simulink model "EQmovSimulink"  (R2013b)
settings: Solver=ode3  StartTime=0.0  StopTime=20  FixedStep=1/1200  RelTol=1e-3
undefined symbols (not defined in the file or in its folder): sigbuilder_block
libraries: simulink_extras x1
settings Model: Creator=AGSilva  LastModifiedBy=AGSilva
settings DataIOCC: LimitDataPoints=off  SaveFormat=StructureWithTime  SaveOutput=off  SignalLogging=off  SaveTime=off

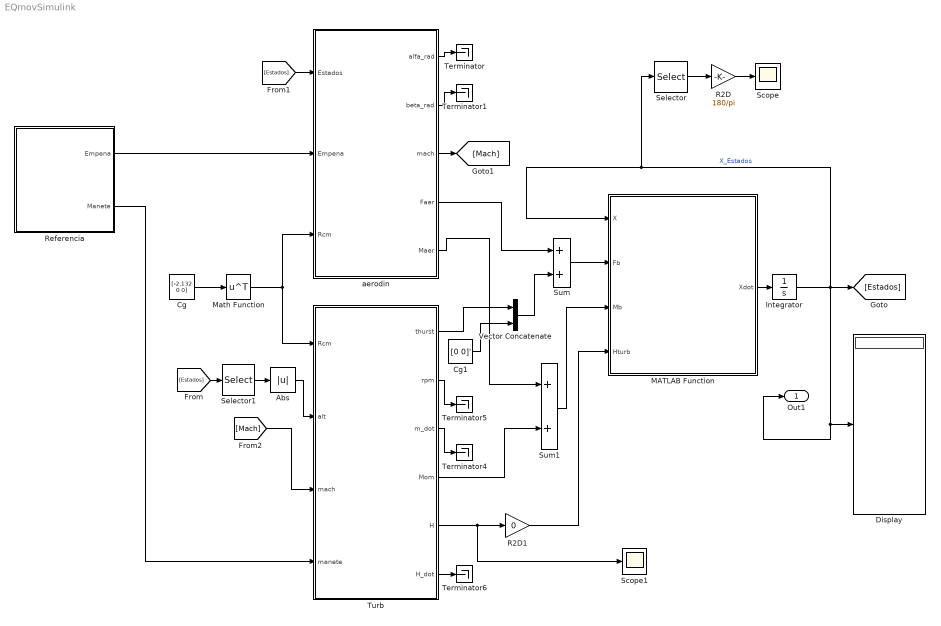
== system EQmovSimulink ==
  Abs : Abs
  Cg : Constant  Value="[-2.132           0           0]"
  Cg1 : Constant  Value=[0 0]'
  Display : Display
  Integrator : Integrator  InitialCondition="[156.55944     0.15954293      33.001765              0     0.20775238              0              0              0              0              0              0          -3000]"
  MATLAB Function : MATLAB Function  TreatAsAtomicUnit=on
  Math Function : Math  Operator=transpose  SaturateOnIntegerOverflow=on
  R2D : Gain  Gain=180/pi
  R2D1 : Gain  Gain=0
  Referencia : Subsystem
  Scope : Scope
  Scope1 : Scope
      settings: SaveName=ScopeData2
  Selector : Selector  InputPortWidth=12  IndexOptions=Index vector (dialog)  Indices=[4]  OutputSizes=1
  Selector1 : Selector  InputPortWidth=12  IndexOptions=Index vector (dialog)  Indices=[12]  OutputSizes=1
  Sum : Sum
  Sum1 : Sum
  Terminator{,1,4..6} (5 alike) : Terminator
  Turb : Subsystem  TreatAsAtomicUnit=on
  Vector Concatenate : Concatenate
  aerodin : Subsystem  TreatAsAtomicUnit=on
  Out1 : Outport
  wires:
  MATLAB Function/1(Xdot) -> Integrator/1
  Integrator/1 -> Selector/1, MATLAB Function/1(X), [Estados], Out1/1, Display/1  "X_Estados"
  Sum1/1 -> MATLAB Function/3(Mb)
  Sum/1 -> MATLAB Function/2(Fb)
  aerodin/1(alfa_rad) -> Terminator/1
  aerodin/2(beta_rad) -> Terminator1/1
  aerodin/3(mach) -> [Mach]
  [Estados] -> Selector1/1
  [Estados] -> aerodin/1(Estados)
  Selector/1 -> R2D/1
  R2D/1 -> Scope/1
  aerodin/5(Maer) -> Sum1/1
  Referencia/1(Empena) -> aerodin/2(Empena)
  Cg/1 -> Math Function/1
  [Mach] -> Turb/3(mach)
  Turb/2(rpm) -> Terminator5/1
  Turb/3(m_dot) -> Terminator4/1
  Turb/4(Mom) -> Sum1/2
  Turb/5(H) -> Scope1/1, R2D1/1
  Turb/6(H_dot) -> Terminator6/1
  Abs/1 -> Turb/2(alt)
  Selector1/1 -> Abs/1
  Referencia/2(Manete) -> Turb/4(manete)
  R2D1/1 -> MATLAB Function/4(Hturb)
  aerodin/4(Faer) -> Sum/1
  Vector Concatenate/1 -> Sum/2
  Turb/1(thurst) -> Vector Concatenate/1
  Cg1/1 -> Vector Concatenate/2
  Math Function/1 -> aerodin/3(Rcm), Turb/1(Rcm)

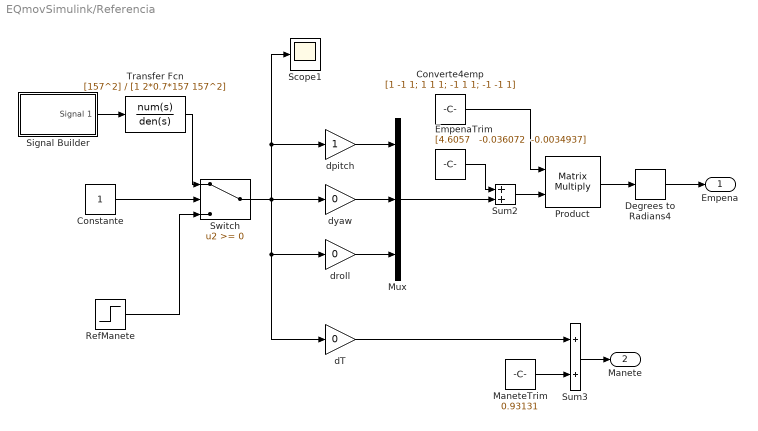
== system EQmovSimulink/Referencia ==
  Constante : Constant
  Converte4emp : Constant  Value=[1 -1 1; 1 1 1; -1 1 1; -1 -1 1]
  Degrees to Radians4 : simulink_extras/Transformations/Degrees to Radians
  EmpenaTrim : Constant  Value="[4.6057   -0.036072  -0.0034937]"
  ManeteTrim : Constant  Value=0.93131
  Mux : Mux  Inputs=3
  Product : Product  Multiplication=Matrix(*)
  RefManete : Step  After=0.05  SampleTime=0
  Scope1 : Scope
  Signal Builder : Subsystem  Tag=STV Subsys  LoadFcn=sigbuilder_block('load');  StartFcn=sigbuilder_block('start');  StopFcn=sigbuilder_block('stop');  ClipboardFcn=sigbuilder_block('clipboard');  mask(Sigbuilder block){}
      mask help: Sigbuilder GUI
      mask init:
      | if ~strcmp(get_param(bdroot(gcbh),'SimulationStatus'),'stopped') tuvar = sigbuilder_block('maskInit'); end
      settings: CopyFcn=sigbuilder_block('copy');  DeleteFcn=sigbuilder_block('delete');  ModelCloseFcn=sigbuilder_block('modelClose');  PreSaveFcn=sigbuilder_block('preSave');  PauseFcn=sigbuilder_block('pause')  ContinueFcn=sigbuilder_block('continue')  NameChangeFcn=sigbuilder_block('namechange');  OpenFcn=sigbuilder_block('open',[6 28.5 1248 693 ]);  CloseFcn=sigbuilder_block('close');
      mask Display: plot(0,0,100,100,[10,10,40,40,10],[80,20,20,80,80],[40,10],[50,50], [40,27,10],[65,72,56],[40,25,25,10],[28,28,43,43]);
  Sum2 : Sum
  Sum3 : Sum
  Switch : Switch
  Transfer Fcn : TransferFcn  Numerator=[157^2]  Denominator=[1 2*0.7*157 157^2]
  dT : Gain  Gain=0
  dpitch : Gain
  droll : Gain  Gain=0
  dyaw : Gain  Gain=0
  Empena : Outport
  Manete : Outport  Port=2
  wires:
  Converte4emp/1 -> Product/1
  Product/1 -> Degrees to Radians4/1
  Degrees to Radians4/1 -> Empena/1
  RefManete/1 -> Switch/3
  droll/1 -> Mux/3
  Signal Builder/1(Signal 1) -> Transfer Fcn/1
  dpitch/1 -> Mux/1
  dyaw/1 -> Mux/2
  Mux/1 -> Sum2/2
  EmpenaTrim/1 -> Sum2/1
  Sum2/1 -> Product/2
  Switch/1 -> dT/1, droll/1, dpitch/1, Scope1/1, dyaw/1
  Sum3/1 -> Manete/1
  dT/1 -> Sum3/1
  ManeteTrim/1 -> Sum3/2
  Transfer Fcn/1 -> Switch/1
  Constante/1 -> Switch/2

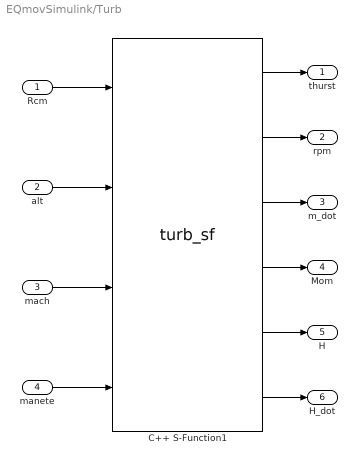
== system EQmovSimulink/Turb ==
  Rcm : Inport
  alt : Inport  Port=2
  mach : Inport  Port=3
  manete : Inport  Port=4
  C++ S-Function1 : S-Function  FunctionName=turb_sf  EnableBusSupport=off
  thurst : Outport
  rpm : Outport  Port=2
  m_dot : Outport  Port=3
  Mom : Outport  Port=4
  H : Outport  Port=5
  H_dot : Outport  Port=6
  wires:
  Rcm/1 -> C++ S-Function1/1
  alt/1 -> C++ S-Function1/2
  mach/1 -> C++ S-Function1/3
  manete/1 -> C++ S-Function1/4
  C++ S-Function1/6 -> H_dot/1
  C++ S-Function1/5 -> H/1
  C++ S-Function1/1 -> thurst/1
  C++ S-Function1/2 -> rpm/1
  C++ S-Function1/3 -> m_dot/1
  C++ S-Function1/4 -> Mom/1

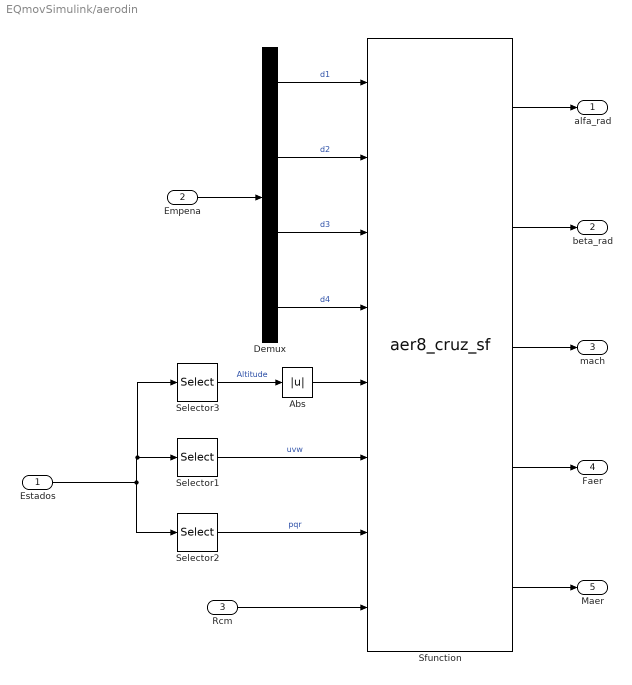
== system EQmovSimulink/aerodin ==
  Estados : Inport
  Empena : Inport  Port=2
  Rcm : Inport  Port=3
  Abs : Abs
  Demux : Demux
  Selector1 : Selector  InputPortWidth=12  IndexOptions=Index vector (dialog)  Indices=[1 2 3]  OutputSizes=1
  Selector2 : Selector  InputPortWidth=12  IndexOptions=Index vector (dialog)  Indices=[7 8 9]  OutputSizes=1
  Selector3 : Selector  InputPortWidth=12  IndexOptions=Index vector (dialog)  Indices=[12]  OutputSizes=1
  Sfunction : S-Function  FunctionName=aer8_cruz_sf  EnableBusSupport=off
  alfa_rad : Outport
  beta_rad : Outport  Port=2
  mach : Outport  Port=3
  Faer : Outport  Port=4
  Maer : Outport  Port=5
  wires:
  Selector1/1 -> Sfunction/6  "uvw"
  Empena/1 -> Demux/1
  Selector3/1 -> Abs/1  "Altitude"
  Abs/1 -> Sfunction/5
  Demux/1 -> Sfunction/1  "d1"
  Demux/2 -> Sfunction/2  "d2"
  Demux/3 -> Sfunction/3  "d3"
  Demux/4 -> Sfunction/4  "d4"
  Selector2/1 -> Sfunction/7  "pqr"
  Estados/1 -> Selector3/1, Selector1/1, Selector2/1
  Sfunction/1 -> alfa_rad/1
  Sfunction/2 -> beta_rad/1
  Sfunction/3 -> mach/1
  Sfunction/4 -> Faer/1
  Sfunction/5 -> Maer/1
  Rcm/1 -> Sfunction/8

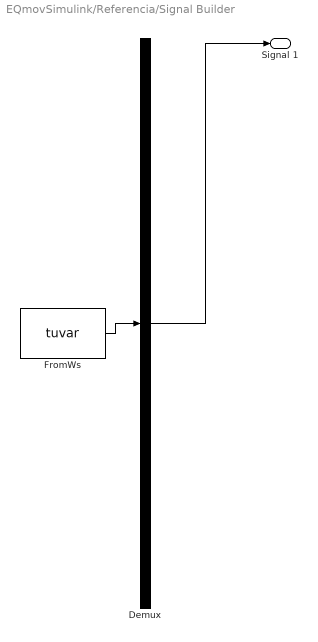
== system EQmovSimulink/Referencia/Signal Builder ==
  Demux : Demux  Tag=STV Demux  Outputs=1
  FromWs : FromWorkspace  Tag=STV FromWs  VariableName=tuvar  SampleTime=0
      SigBuilderData=|
      | common.afterFinalStr = 'Extrapolate'
      | common.sampleTime = 0
      | dataSet.timeRange = [0 10]
      | dataSet.name = 'Group 1'
      | sbobj.Groups.Name = 'Group 1'
      | sbobj.Groups.Signals.Name = 'Signal 1'
      | sbobj.Groups.Signals.XData = [0 1 1 1.25 1.25 1.5 1.5 10]
      | sbobj.Groups.Signals.YData = [0 0 1 1 -1 -1 0 0]
  Signal 1 : Outport  Tag=STV Outport
  wires:
  Demux/1 -> Signal 1/1
  FromWs/1 -> Demux/1

== matlab function EQmovSimulink/MATLAB Function ==
  data: X input; Fb input; Mb input; Aux_Modelo parameter; Hturb input; Xdot output
function Xdot = EQmovSimulink(X, Fb, Mb, Aux_Modelo, Hturb)

p = X(7);
q = X(8);
r = X(9);

W = [p q r]';

mass = Aux_Modelo.Massa;
J = Aux_Modelo.Inercia;

phi = X(4);
theta = X(5);
psi = X(6);

cphi = cos(phi);
sphi = sin(phi);
ctheta = cos(theta);
stheta = sin(theta);
cpsi = cos(psi);
spsi = sin(psi);
    
% Lewis página 46

g = 9.8066;
G_vet = [0; 0; g];

Cnb = [         ctheta*cpsi             ctheta*spsi                 -stheta
        -cphi*spsi+sphi*stheta*cpsi  cphi*cpsi+sphi*stheta*spsi   sphi*ctheta
         sphi*spsi+cphi*stheta*cpsi -sphi*cpsi+cphi*stheta*spsi   cphi*ctheta];
     
Cbn = Cnb';

OMEGA = [ 0 -r  q
          r  0 -p
         -q  p  0];
     
ETA = [ 1  stheta*sphi/ctheta  stheta*cphi/ctheta
        0           cphi                -sphi
        0       sphi/ctheta         cphi/ctheta];
    
% Force Equation
V_dot = (Fb/mass) - OMEGA*X(1:3) + Cnb*G_vet;

% Atitude Equation;
Euler_dot = ETA*W;

% Momento Equation
% Hturb = [0 0 0]';

% W_dot = J\(-OMEGA*(J*W) + Mb ) - OMEGA*Hturb;
W_dot = J\(-OMEGA*(J*W + Hturb) + Mb );

%Navigation Equation
Pn_dot = Cbn*X(1:3);

Xdot = [V_dot; Euler_dot; W_dot; Pn_dot];

end
